simulink model "MAXM8"  (R2020a)
settings: Solver=FixedStepAuto  StartTime=0.0  StopTime=10.0  RelTol=1e-3
values from neighbouring files (symbols this model uses):
  MAXM8_altitude_variance = (2.5*1.7)^2    (= 18.0625)    [configure_simulation.m]    (also in test_kalman.m)
  MAXM8_sample_rate = 10    [configure_simulation.m]
  MAXM8_velocity_variance = (0.05)^2    (= 0.0025)    [configure_simulation.m]    (also in test_kalman.m)
settings Model: Creator=Philip  LastModifiedBy=Philip

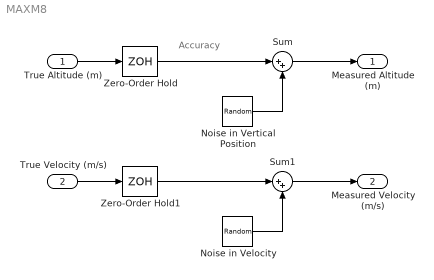
== system MAXM8 ==
  note: Accuracy
  True Altitude (m) : Inport
  True Velocity (m/s) : Inport  Port=2
  Noise in Velocity : RandomNumber  Variance=MAXM8_velocity_variance  Seed=100  SampleTime=1/MAXM8_sample_rate
  Noise in Vertical Position : RandomNumber  Variance=MAXM8_altitude_variance  Seed=10  SampleTime=1/MAXM8_sample_rate
  Sum : Sum  Inputs=|++
  Sum1 : Sum  Inputs=|++
  Zero-Order Hold : ZeroOrderHold  SampleTime=1/MAXM8_sample_rate
  Zero-Order Hold1 : ZeroOrderHold  SampleTime=1/MAXM8_sample_rate
  Measured Altitude (m) : Outport
  Measured Velocity (m/s) : Outport  Port=2
  wires:
  True Altitude (m)/1 -> Zero-Order Hold/1
  Noise in Vertical Position/1 -> Sum/2
  True Velocity (m/s)/1 -> Zero-Order Hold1/1
  Noise in Velocity/1 -> Sum1/2
  Sum1/1 -> Measured Velocity (m/s)/1
  Sum/1 -> Measured Altitude (m)/1
  Zero-Order Hold/1 -> Sum/1
  Zero-Order Hold1/1 -> Sum1/1
